simulink subsystem "Throttle_Passthrough"  (R2023b)
settings: Solver=VariableStepAuto  StartTime=0.0  StopTime=50  RelTol=1e-3
libraries: simulink x1
settings Model: DefaultTestHarness=LVSS_EN_Harness1  Creator=diego  LastModifiedBy=nickj

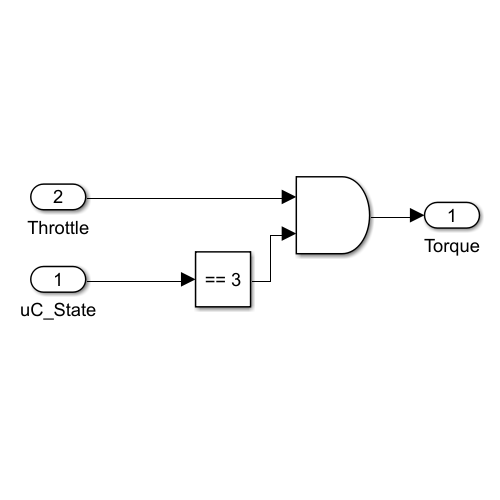
[thumbnail: Simulink's stored preview of the top-level diagram]
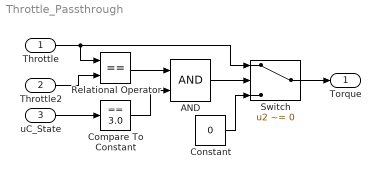
== system Throttle_Passthrough ==
  Throttle : Inport
  Throttle2 : Inport  Port=2
  uC_State : Inport  Port=3
  AND : Logic  IconShape=distinctive  AllPortsSameDT=off  OutDataTypeStr=boolean
  Compare To Constant : simulink/Logic and Bit Operations/Compare To Constant  relop===  const=3.0  OutDataTypeStr=boolean
  Constant : Constant  Value=0
  Relational Operator : RelationalOperator  Operator===  OutDataTypeStr=boolean  RndMeth=Simplest  InputSameDT=off
  Switch : Switch  Criteria=u2 ~= 0  SaturateOnIntegerOverflow=off  InputSameDT=off
  Torque : Outport
  wires:
  uC_State/1 -> Compare To Constant/1
  Relational Operator/1 -> AND/1
  Compare To Constant/1 -> AND/2
  Switch/1 -> Torque/1
  AND/1 -> Switch/2
  Constant/1 -> Switch/3
  Throttle/1 -> Switch/1, Relational Operator/1
  Throttle2/1 -> Relational Operator/2
